simulink model "Diagrama_entrada_triangular_tempo_discretizado"  (R2022b)
settings: Solver=VariableStepAuto  StartTime=0.0  StopTime=10  RelTol=1e-3
values from neighbouring files (symbols this model uses):
  betha = n    (= 7)    [Q1.m]    (also in Q2_raizes.m = 2.85714285714)
  betha_e = 20/n    (= 2.85714285714)    [Q2_raizes.m]
  g = 9.8    [Q2_raizes.m]
  Jm = n    (= 7)    [Q2_raizes.m]
  Kb = 0.1*n    (= 0.7)    [Q2_raizes.m]
  Ki = 20/n    (= 2.85714285714)    [Q2_raizes.m]
  La = 0.1*n    (= 0.7)    [Q2_raizes.m]
  m = sqrt(1/n)    [Q2_raizes.m]
  Ra = 20/n    (= 2.85714285714)    [Q2_raizes.m]
libraries: simulink x1
settings Model: Creator=kaiqu  LastModifiedBy=kaiqu

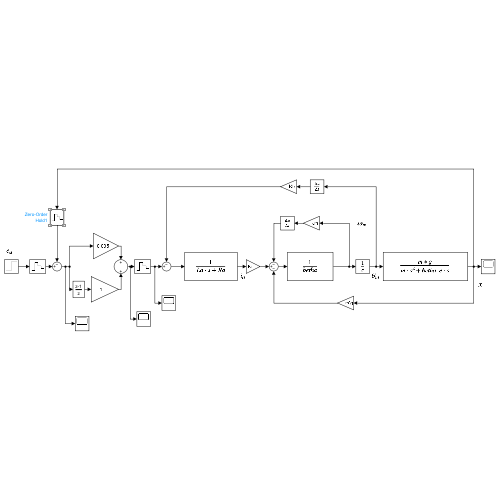
[thumbnail: Simulink's stored preview of the top-level diagram]
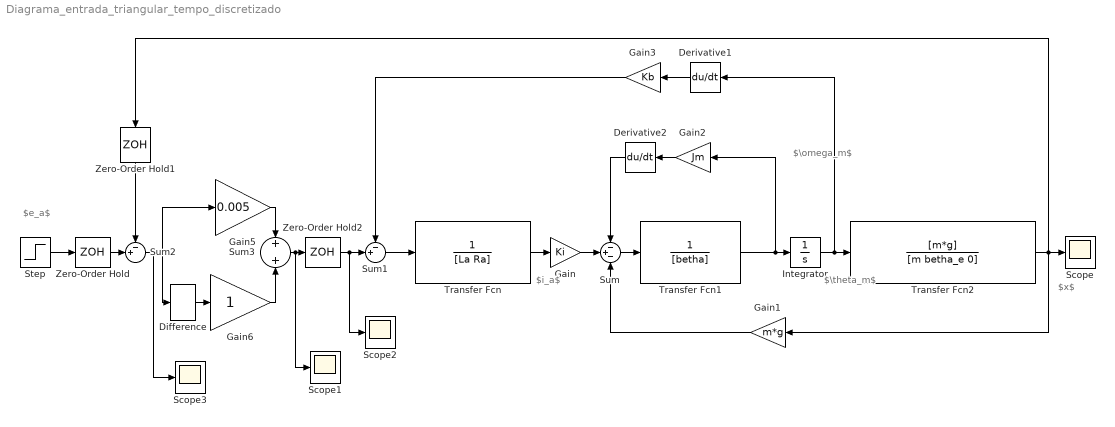
== system Diagrama_entrada_triangular_tempo_discretizado ==
  note: $i_a$
  note: $e_a$
  note: $\omega_m$
  note: $\theta_m$
  note: $x$
  Derivative1 : Derivative
  Derivative2 : Derivative
  Difference : simulink/Discrete/Difference  ICPrevInput=0.0  OutMin=[]  OutMax=[]  OutDataType=fixdt(1, 16)  OutScaling=2^-10  DoSatur=off
  Gain : Gain  Gain=Ki
  Gain1 : Gain  Gain=m*g
  Gain2 : Gain  Gain=Jm
  Gain3 : Gain  Gain=Kb
  Gain5 : Gain  Gain=0.005
  Gain6 : Gain
  Integrator : Integrator
  Scope{,1..3} (4 alike) : Scope
  Step : Step  Time=0  SampleTime=0
  Sum : Sum  Inputs=-+-
  Sum1 : Sum  Inputs=-+|
  Sum2 : Sum  Inputs=-+|
  Sum3 : Sum  Inputs=+|+
  Transfer Fcn : TransferFcn  Denominator=[La Ra]
  Transfer Fcn1 : TransferFcn  Denominator=[betha]
  Transfer Fcn2 : TransferFcn  Numerator=[m*g]  Denominator=[m betha_e 0]
  Zero-Order Hold : ZeroOrderHold  SampleTime=0.1
  Zero-Order Hold1 : ZeroOrderHold  SampleTime=0.1
  Zero-Order Hold2 : ZeroOrderHold  SampleTime=0.1
  wires:
  Derivative1/1 -> Gain3/1
  Derivative2/1 -> Sum/1
  Gain/1 -> Sum/2
  Sum2/1 -> Scope3/1, Difference/1, Gain5/1
  Gain1/1 -> Sum/3
  Gain5/1 -> Sum3/1
  Gain3/1 -> Sum1/1
  Difference/1 -> Gain6/1
  Transfer Fcn1/1 -> Integrator/1, Gain2/1
  Transfer Fcn/1 -> Gain/1
  Gain2/1 -> Derivative2/1
  Sum1/1 -> Transfer Fcn/1
  Integrator/1 -> Derivative1/1, Transfer Fcn2/1
  Sum/1 -> Transfer Fcn1/1
  Transfer Fcn2/1 -> Zero-Order Hold1/1, Gain1/1, Scope/1
  Gain6/1 -> Sum3/2
  Zero-Order Hold/1 -> Sum2/2
  Step/1 -> Zero-Order Hold/1
  Zero-Order Hold1/1 -> Sum2/1
  Sum3/1 -> Scope1/1, Zero-Order Hold2/1
  Zero-Order Hold2/1 -> Scope2/1, Sum1/2
